simulink model "system4"  (R2018b)
settings: Solver=VariableStepAuto  StartTime=0.0  StopTime=10  RelTol=1e-3
libraries: cstblocks x5, simulink x1
settings Model: Creator=Abraham Pérez  LastModifiedBy=Abraham Pérez

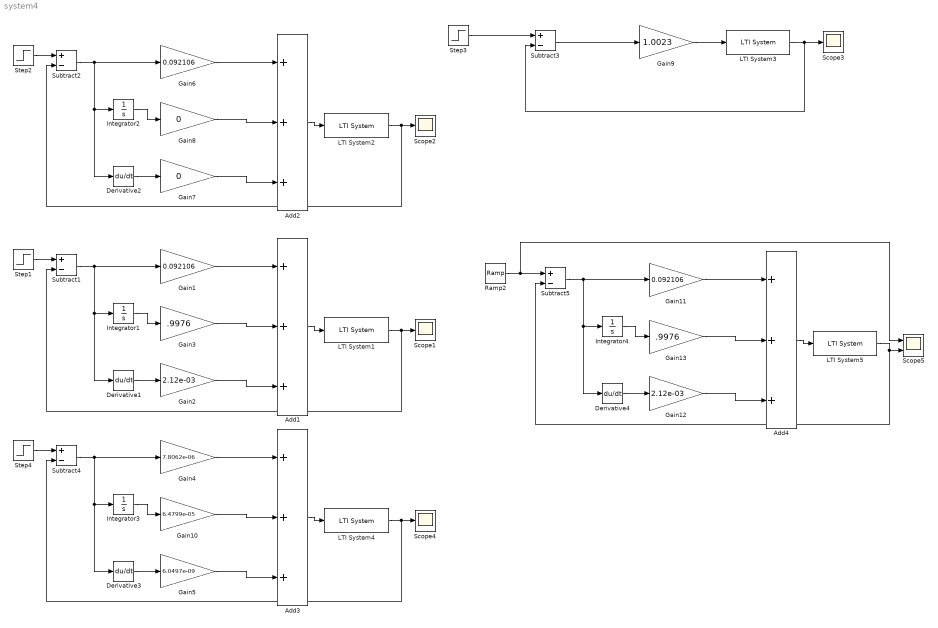
== system system4 ==
  Add{1..4} (4 alike) : Sum  Inputs=+++
  Derivative{1..4} (4 alike) : Derivative
  Gain1 : Gain  Gain=0.092106
  Gain10 : Gain  Gain=6.4799e-05
  Gain11 : Gain  Gain=0.092106
  Gain12 : Gain  Gain=2.12e-03
  Gain13 : Gain  Gain=.9976
  Gain2 : Gain  Gain=2.12e-03
  Gain3 : Gain  Gain=.9976
  Gain4 : Gain  Gain=7.8062e-06
  Gain5 : Gain  Gain=6.0497e-09
  Gain6 : Gain  Gain=0.092106
  Gain7 : Gain  Gain=0
  Gain8 : Gain  Gain=0
  Gain9 : Gain  Gain=1.0023
  Integrator{1..4} (4 alike) : Integrator
  LTI System{1..5} (5 alike) : cstblocks/LTI System  sys=G4  IC=[]
  Ramp2 : simulink/Sources/Ramp  slope=1  start=0  InitialOutput=17
  Scope{1..4} (4 alike) : Scope
  Scope5 : Scope  NumInputPorts=2
  Step1 : Step  Time=0  After=9  SampleTime=0
  Step2 : Step  Time=0  After=9  SampleTime=0
  Step3 : Step  Time=0  SampleTime=0
  Step4 : Step  Time=0  After=9  SampleTime=0
  Subtract{1..5} (5 alike) : Sum  Inputs=+-
  wires:
  LTI System3/1 -> Subtract3/2, Scope3/1
  LTI System2/1 -> Subtract2/2, Scope2/1
  Step3/1 -> Subtract3/1
  Subtract2/1 -> Derivative2/1, Integrator2/1, Gain6/1
  Gain9/1 -> LTI System3/1
  Integrator2/1 -> Gain8/1
  Add2/1 -> LTI System2/1
  Gain8/1 -> Add2/2
  Step2/1 -> Subtract2/1
  Gain6/1 -> Add2/1
  Subtract3/1 -> Gain9/1
  Derivative2/1 -> Gain7/1
  Gain7/1 -> Add2/3
  LTI System1/1 -> Subtract1/2, Scope1/1
  Gain2/1 -> Add1/3
  Derivative1/1 -> Gain2/1
  Gain1/1 -> Add1/1
  Step1/1 -> Subtract1/1
  Subtract1/1 -> Derivative1/1, Integrator1/1, Gain1/1
  Integrator1/1 -> Gain3/1
  Gain3/1 -> Add1/2
  Add1/1 -> LTI System1/1
  Gain10/1 -> Add3/2
  LTI System4/1 -> Subtract4/2, Scope4/1
  Gain4/1 -> Add3/1
  Add3/1 -> LTI System4/1
  Gain5/1 -> Add3/3
  Integrator3/1 -> Gain10/1
  Step4/1 -> Subtract4/1
  Subtract4/1 -> Derivative3/1, Integrator3/1, Gain4/1
  Derivative3/1 -> Gain5/1
  Gain13/1 -> Add4/2
  LTI System5/1 -> Subtract5/2, Scope5/2
  Gain11/1 -> Add4/1
  Add4/1 -> LTI System5/1
  Gain12/1 -> Add4/3
  Integrator4/1 -> Gain13/1
  Subtract5/1 -> Derivative4/1, Integrator4/1, Gain11/1
  Derivative4/1 -> Gain12/1
  Ramp2/1 -> Scope5/1, Subtract5/1
